simulink library "Wall_out"  (R2018b)
settings: Solver=ode45  StartTime=0.0  StopTime=10.0  RelTol=1e-3  EnableMultiTasking=on
libraries: carnot x3
settings Model: Creator=lena.frank  LastModifiedBy=P41573
settings DataIOCC: LimitDataPoints=on  SaveFormat=Array  SignalLoggingSaveFormat=ModelDataLogs
settings OptimizationCC: ExpressionDepthLimit=2147483647  LifeSpan=inf
settings DebuggingCC: UnderspecifiedInitializationDetection=Classic  MergeDetectMultiDrivingBlocksExec=none  SolverPrmCheckMsg=warning  FcnCallInpInsideContextMsg=warning  StateNameClashWarn=warning  SFUnexpectedBacktrackingDiag=warning  SFNoUnconditionalDefaultTransitionDiag=warning  SFExecutionAtInitializationDiag=none
settings HardwareCC: ProdBitPerPointer=32  ProdBitPerSizeT=32  ProdBitPerPtrDiffT=32  ProdLargestAtomicFloat=None  ProdIntDivRoundTo=Undefined  ProdEndianess=Unspecified  ProdWordSize=32  ProdHWDeviceType=32-bit Generic
settings ModelReferenceCC: PropagateSignalLabelsOutOfModel=off
settings SFSimCC: SimUseLocalCustomCode=off
settings RTWCC: RTWUseLocalCustomCode=off
settings CodeAppCC: StateflowObjectComments=on
settings GRTTargetCC: TargetLangStandard=C89/C90 (ANSI)  GeneratePreprocessorConditionals=Disable all  CombineOutputUpdateFcns=off  GRTInterface=on
settings ConfigComp: CovMetricSettings=dw  CovHtmlReporting=on  CovSaveCumulativeToWorkspaceVar=on  CovSaveSingleToWorkspaceVar=on  CovExternalEMLEnable=off

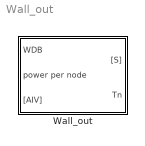
== system Wall_out ==
  Wall_out : Subsystem  mask(outer wall){wallsize=[2.5 5], pos=180, t0=20, d=[0.1 0.38], cond=[0.04 0.79], cwall=[0.28 0.28]*3600, rho=[900 1800], reflectground=0.2, abs_emiss=[0.65 0.97 0.96], tau=1000*3600, dactive=-1}
      mask prompts: wallsize "size of wall [m] [height width]"; pos "azimut (0=south, east = -90)"; t0 "initial temperature [degree centigrade]"; d "thickness of nodes [m] (vector)"; cond "conductivity of nodes [W/(m*K)] (vector)"; cwall "capacity of nodes [J/(kg*K)] (vector)"; rho "density [kg/m^3]"; reflectground "reflection of ground"; abs_emiss "[outer absorption, outer emission, inner emisson]"; tau "time-constant of wall [s]"; dactive "depth of active layer in m from outside (-1, if none)"
      mask help:
      | This is the model of an outer wall of a house.
      | first element of the vector = layer to surrounding
      | last element of the vector = layer to room
      | The azimut may be a scalar or vector with [inclination azimut rotation], see carnot/Weather/Fixed_Surface.
      mask init:
      | if length(pos) == 1
      |     pos = [90  pos 0]; % pos is [inclination azimut rotation]
      | end
      | absorption_out = min(1, max(abs_emiss(1),0));
      | % nodes = length(d);
      | wallsurface = wallsize(1)* wallsize(2);
      | emission_in = abs_emiss(3);
      | emission_out = abs_emiss(2);
      | active = 0;
      | if (dactive>=0) active=1; end
      | 
      | %für Variablen in shaderad
      | wallangle = pos(1);
      | wallazimut = pos(2);
      | wallheight = wallsize(1);
      | wallwidth = wallsize(2);
      mask Help: web(fullfile(path_carnot('help'),'Wall_out.html'),'-helpbrowser')

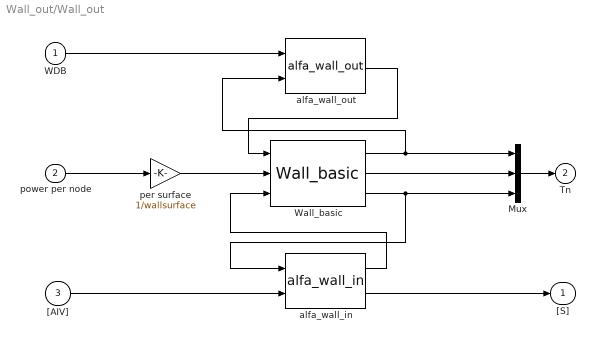
== system Wall_out/Wall_out ==
  WDB : Inport
  power per node : Inport  Port=2
  "[AIV]" : Inport  Port=3
  Mux : Mux  Inputs=3
  Wall_basic : carnot/Basic/Thermal_Models/Wall_basic  tau=tau  t0=t0  d=d  dactive=dactive  cond=cond  cwall=cwall  rho=rho
      settings: SourceProductName=Carnot
  alfa_wall_in : carnot/Basic/Heat_Transfer/alfa_wall_in  active=active  emission_in=emission_in  wallsurface=wallsurface
      settings: SourceProductName=Carnot
  alfa_wall_out : carnot/Basic/Heat_Transfer/alfa_wall_out  pos=pos  absorption_out=absorption_out  emission_out=emission_out  wallsurface=wallsurface
      settings: SourceProductName=Carnot
  per surface : Gain  Gain=1/wallsurface  SaturateOnIntegerOverflow=on  OutDataTypeStr=Inherit: Same as input  ParamDataTypeStr=Inherit: Same as input
  "[S]" : Outport
  Tn : Outport  Port=2
  wires:
  Mux/1 -> Tn/1
  Wall_basic/2 -> Mux/2
  WDB/1 -> alfa_wall_out/1
  power per node/1 -> per surface/1
  per surface/1 -> Wall_basic/2
  alfa_wall_out/1 -> Wall_basic/1
  Wall_basic/1 -> alfa_wall_out/2, Mux/1
  alfa_wall_in/1 -> Wall_basic/3
  Wall_basic/3 -> alfa_wall_in/1, Mux/3
  "[AIV]"/1 -> alfa_wall_in/2
  alfa_wall_in/2 -> "[S]"/1
